simulink model "Sum15"  (Simulink 9.0)
settings: Solver=FixedStepAuto  StartTime=0.0  StopTime=10.0  FixedStep=0.1  RelTol=1e-3  EnableMultiTasking=on
settings Model: SuppressorTable=22 serialization::archive 11 0 6 0 0 0 0 0  Creator=arnaud  LastModifiedBy=hbourbou
settings DataIOCC: LimitDataPoints=on  SaveFormat=Structure  SignalLoggingSaveFormat=ModelDataLogs
settings OptimizationCC: ExpressionDepthLimit=2147483647
settings DebuggingCC: SolverPrmCheckMsg=warning  FcnCallInpInsideContextMsg=warning  StateNameClashWarn=warning
settings GRTTargetCC: GeneratePreprocessorConditionals=Disable all  CombineOutputUpdateFcns=off  GRTInterface=on
settings ConfigComp: CovSFcnEnable=off

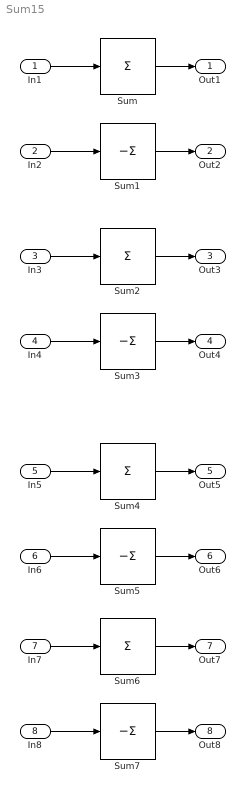
== system Sum15 ==
  In1 : Inport
  In2 : Inport  Port=2
  In3 : Inport  Port=3  PortDimensions=3
  In4 : Inport  Port=4  PortDimensions=3
  In5 : Inport  Port=5  PortDimensions=[2 3]
  In6 : Inport  Port=6  PortDimensions=[2 3]
  In7 : Inport  Port=7  PortDimensions=[2 3]
  In8 : Inport  Port=8  PortDimensions=[2 3]
  Sum : Sum  Inputs=+  CollapseMode=Specified dimension
  Sum1 : Sum  Inputs=-  CollapseMode=Specified dimension
  Sum2 : Sum  Inputs=+  CollapseMode=Specified dimension
  Sum3 : Sum  Inputs=-  CollapseMode=Specified dimension
  Sum4 : Sum  Inputs=+  CollapseMode=Specified dimension
  Sum5 : Sum  Inputs=-  CollapseMode=Specified dimension
  Sum6 : Sum  Inputs=+  CollapseMode=Specified dimension  CollapseDim=2
  Sum7 : Sum  Inputs=-  CollapseMode=Specified dimension  CollapseDim=2
  Out1 : Outport
  Out2 : Outport  Port=2
  Out3 : Outport  Port=3
  Out4 : Outport  Port=4
  Out5 : Outport  Port=5
  Out6 : Outport  Port=6
  Out7 : Outport  Port=7
  Out8 : Outport  Port=8
  wires:
  In1/1 -> Sum/1
  Sum/1 -> Out1/1
  In2/1 -> Sum1/1
  Sum1/1 -> Out2/1
  In3/1 -> Sum2/1
  Sum2/1 -> Out3/1
  In4/1 -> Sum3/1
  Sum3/1 -> Out4/1
  In5/1 -> Sum4/1
  Sum4/1 -> Out5/1
  In6/1 -> Sum5/1
  Sum5/1 -> Out6/1
  In7/1 -> Sum6/1
  Sum6/1 -> Out7/1
  In8/1 -> Sum7/1
  Sum7/1 -> Out8/1
